simulink model "l5"  (R2015a)
settings: Solver=ode45  StartTime=0.0  StopTime=10.0  RelTol=1e-3
undefined symbols (not defined in the file or in its folder): prova_sim_sistema
settings Model: Creator=lezione00  LastModifiedBy=lezione00

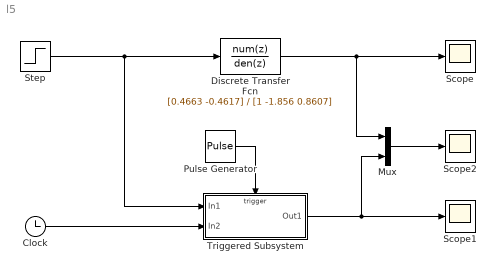
== system l5 ==
  Clock : Clock
  Discrete Transfer Fcn : DiscreteTransferFcn  Numerator=[0.4663 -0.4617]  Denominator=[1 -1.856 0.8607]  SampleTime=0.1
  Mux : Mux  Inputs=2
  Pulse Generator : DiscretePulseGenerator  PulseType=Time based  Period=0.1  PulseWidth=5
  Scope : Scope
  Scope1 : Scope
  Scope2 : Scope
      settings: SaveName=ScopeData2
  Step : Step  SampleTime=0
  Triggered Subsystem : Subsystem  TreatAsAtomicUnit=on
  wires:
  Step/1 -> Triggered Subsystem/1(In1), Discrete Transfer Fcn/1
  Discrete Transfer Fcn/1 -> Mux/1, Scope/1
  Triggered Subsystem/1(Out1) -> Mux/2, Scope1/1
  Clock/1 -> Triggered Subsystem/2(In2)
  Pulse Generator/1 -> Triggered Subsystem/Trigger
  Mux/1 -> Scope2/1

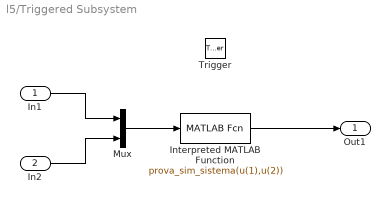
== system l5/Triggered Subsystem ==
  In1 : Inport
  In2 : Inport  Port=2
  Trigger : TriggerPort
  Interpreted MATLAB Function : MATLABFcn  MATLABFcn=prova_sim_sistema(u(1),u(2))
  Mux : Mux  Inputs=2
  Out1 : Outport
  wires:
  Interpreted MATLAB Function/1 -> Out1/1
  In1/1 -> Mux/1
  Mux/1 -> Interpreted MATLAB Function/1
  In2/1 -> Mux/2
